simulink model "practica1_ej2_simulink"  (R2023b)
settings: Solver=VariableStepAuto  StartTime=0.0  StopTime=10.0  RelTol=1e-3
model workspace (MAT data in the model file):
  C = 0.001
  L = 1
  R = 1000
settings Model: Creator=Máximo  LastModifiedBy=Máximo

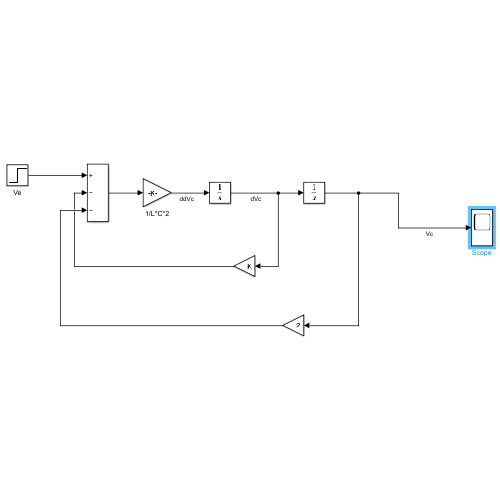
[thumbnail: Simulink's stored preview of the top-level diagram]
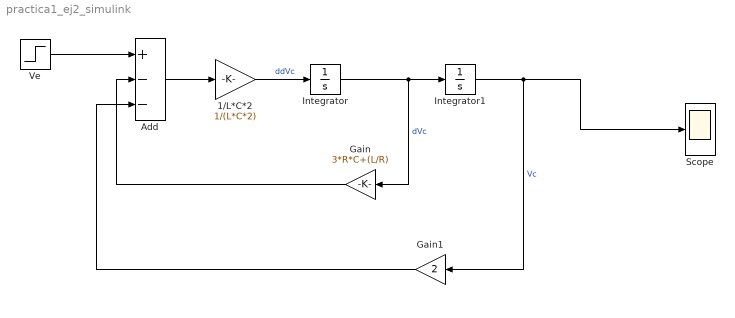
== system practica1_ej2_simulink ==
  1/L*C*2 : Gain  Gain=1/(L*C*2)
  Add : Sum  Inputs=+--
  Gain : Gain  Gain=3*R*C+(L/R)
  Gain1 : Gain  Gain=2
  Integrator : Integrator
  Integrator1 : Integrator
  Scope : Scope
  Ve : Step  Time=0  Before=1  SampleTime=0
  wires:
  Ve/1 -> Add/1
  Add/1 -> 1/L*C*2/1
  1/L*C*2/1 -> Integrator/1  "ddVc"
  Integrator/1 -> Gain/1, Integrator1/1  "dVc"
  Integrator1/1 -> Gain1/1, Scope/1  "Vc"
  Gain1/1 -> Add/3
  Gain/1 -> Add/2
